simulink model "main_sim"  (R2025b)
settings: Solver=VariableStepAuto  StartTime=0.0  StopTime=6  RelTol=1e-3
model workspace (MAT data in the model file):
  Axy = [0  0  0  0; 0  0  0  0; 0  0  0  0; 0  0  0  0]
  Axz = [0  0  1  0; 0  0  0  1; 0  -11.8453251738  0  0; 0  6.95008459918  0  0]
  Ayz = [0  0  1  0; 0  0  0  1; 0  -11.8453251738  0  0; 0  6.95008459918  0  0]
  Bxy = [0  0  0  0; 0  0  0  0; 0  0  0  0; 0  0  0  0]
  Bxz = [0; 0; 9.84767991023; -1.08649077682]
  Byz = [0; 0; 9.84767991023; -1.08649077682]
  Cxy = [0  0  0  0; 0  0  0  0; 0  0  0  0; 0  0  0  0]
  Cxz = [1  0  0  0; 0  1  0  0; 0  0  1  0; 0  0  0  1]
  Cyz = [1  0  0  0; 0  1  0  0; 0  0  1  0; 0  0  0  1]
  Dxy = [0  0  0  0; 0  0  0  0; 0  0  0  0; 0  0  0  0]
  Dxz = [0; 0; 0; 0]
  Dyz = [0; 0; 0; 0]
  ICxy = [0; 0; 0; 0]
  ICxz = [0; 0.3; 0; -0.7]
  ICyz = [0; 0.3; 0; -0.7]
  ptorque = [0 0 0]
  vtorque = [0; 0; 0]
libraries: sim3dlib x7
settings Model: PacingRate=0.400000  Creator=rtsto  LastModifiedBy=rtsto

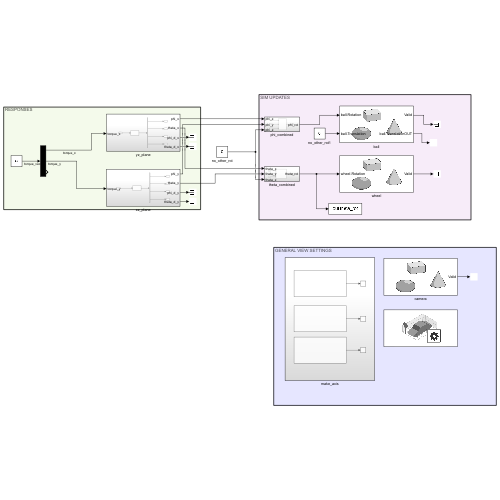
[thumbnail: Simulink's stored preview of the top-level diagram]
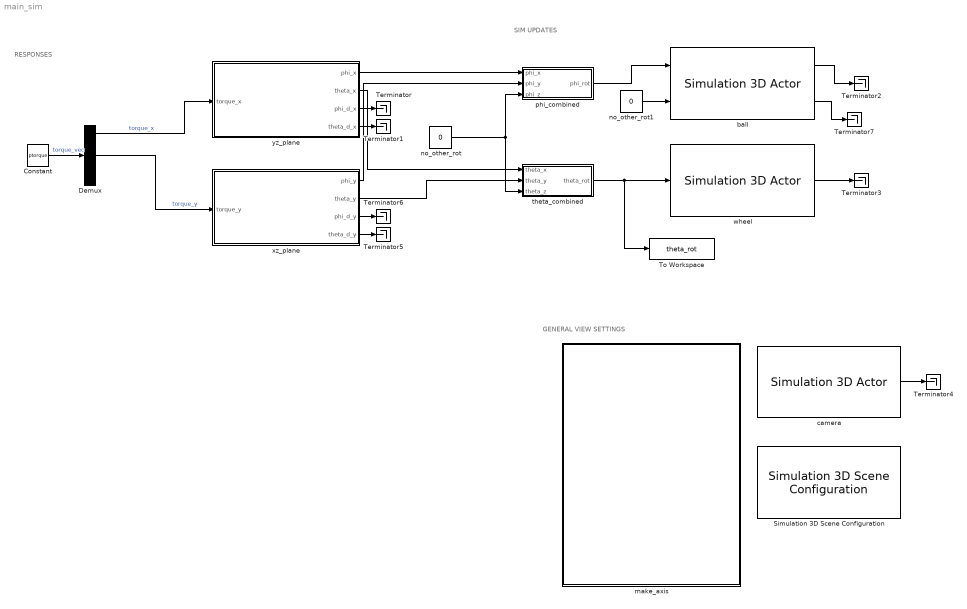
== system main_sim ==
  note: SIM UPDATES
  note: RESPONSES
  note: GENERAL VIEW SETTINGS
  Constant : Constant  Value=ptorque
  Demux : Demux  Outputs=3
  Simulation 3D Scene Configuration : sim3dlib/Simulation 3D Scene Configuration  Priority=0  ProjectFormat=Default Scenes  SceneDesc=Empty scene  ProjectName=C:\Program Files\MATLAB\R2025b\toolbox\shared\sim3d_projects\automotive_project_windows\UE\WindowsNoEditor\VehicleSimulation.exe  ScenePath=/Game/Maps/HwStrght  EnableOpenDRIVE=off  vehTagList={'Custom';'MainScene';'Scene Origin';'Viewpoint1';'World';'ball';'camera';'wheel';'x_axis';'y_axis';'z_axis'}  vehTag=MainScene  AttachedCameraRelativeTranslation=[0 0 0]  FreeCameraDefaultInitialTranslation=[-6, 0, 2]  AttachedCameraRelativeRotation=[0 0 0]  FreeCameraDefaultInitialRotation=[0, -15, 0]  ViewpointName=MainScene  FreeCameraInitialTranslation=[0 0 0]  ViewpointTranslation=[0 0 0]  FreeCameraInitialRotation=[0 0 0]  ViewpointRotation=[0 0 0]  OpVisEn=off  Ts=.02  EnableWindow=on  EnableRemoteAccess=off  EnableWeather=off  SunAzimuth=90  SunAltitude=40.0  EnableGeospatialSun=off  Latitude=0  Longitude=0  Date=2023-01-01  Time=10:30:00  GeoTimeZone=-5.0  SunDaylightSaving=off  wind=1  clouds=10  EnableVolumetricClouds=off  CloudCoverage=0  CloudAltitude=6  fog=0  rain=0  RaindropsEffect=off  SnowDensity=0  EnableGeospatial=off  TilesetSource=Earth terrain  UseTrueOrigin=off  OriginHeight=200  OriginLatitude=40.744652  OriginLongitude=-73.988864  MapStyle=Aerial  AdditionalAssetIDs=[]  UseAdvancedSunSky=off  SolarTime=11  TimeZone=-5  Day=21  Month=9  Year=2022  UseDaylightSavingTime=on  DSTStartDay=10  DSTStartMonth=3  DSTEndDay=3  DSTEndMonth=11  DSTSwitchHour=2  sensorTag=MainCamera1  sensorId=1  sensorName=MainCamera1  mountLoc=Origin  offsetFlag=off  tmountOffset=[0, 0, 0]  rmountOffset=[0, 0, 0]  HorizontalResolution=1280  VerticalResolution=720  HorizontalFOV=60  mountPoint=[0 0 0]  mountOrientation=[0 0 0]  aMode=5  ID=1  GeoTrigger=Inactive  ViewNameList={'Custom', 'World', 'MainScene', 'Viewpoint1'}  ViewTranslationList="{'[0 0 0]', '[0 0 0]', '[0 0 0]', '[-4  4  2]'}"  ViewRotationList="{'[0 0 0]', '[0 0 0]', '[0 0 0]', '[0        -22.5          -45]'}"
      settings: LibrarySourceBlock=sl3dlib/Simulation 3D/Environment/Simulation 3D Scene Configuration
  Terminator{,1..7} (8 alike) : Terminator
  To Workspace : ToWorkspace  VariableName=theta_rot  SampleTime=-1
  ball : sim3dlib/Simulation 3D Actor  Priority=1  ActorName=ball  ParentName=Scene Origin  Operation=Create at setup  InitScriptText=|  SampleTime=-1  Translation=single([0 0 0])  Rotation=single([0 0 0])  Scale=single([1 1 1])  InputsText=ball.Rotation ball.Translation  OutputsText=ball.Translation  aMode=5  ActorTag=ball  ActorType=Sim3dActor  ID=C
      | % BALL LOADING
      |     ball = sim3d.Actor(ActorName='ball', ...
      |         Mobility=sim3d.utils.MobilityTypes.Movable);
      |     load(ball, "ball.stl");
      |     diameter = 12.5; % raw
      |     scale = 0.1; % raw
      |     
      |     radius = scale*diameter/2; %scaled
      |     ball.Scale = scale*[1, 1, 1]; % NOTE: won't change in 'transform' tab
      |     ball.Translation = [0 -radius -radius];
      |     ball.Rotation = [0, pi/2, -pi/2]; % rad
      |     
      |     ball.Physics = false;
      |     ball.Collisions = true;
      |     
      |     ball.Color = [1 0 0];
      |     ball.Metallic = 0.1; % not at all
      |     ball.Shininess = 0; % not at all
      |     World.add(ball, Actor);
  camera : sim3dlib/Simulation 3D Actor  Priority=1  ActorName=camera  ParentName=Scene Origin  Operation=Create at setup  InitScriptText=|  SampleTime=-1  Translation=[0 0 0]  Rotation=[0 0 0]  Scale=[1 1 1]  aMode=5  ActorTag=camera  ActorType=Sim3dActor  ID=C
      | pos = [-4, 4, 2];
      | rot = [0, -22.5*pi/180, -45*pi/180];
      | camera = createViewport(World, ...
      |     Translation=pos, Rotation=rot);
  make_axis : Subsystem
  no_other_rot : Constant  Value=0  OutDataTypeStr=Inherit: Inherit via back propagation
  no_other_rot1 : Constant  Value=0  OutDataTypeStr=Inherit: Inherit via back propagation
  phi_combined : Subsystem
  theta_combined : Subsystem
  wheel : sim3dlib/Simulation 3D Actor  Priority=1  ActorName=wheel  ParentName=Scene Origin  Operation=Create at setup  InitScriptText=|  SampleTime=-1  Translation=single([0 0 0])  Rotation=single([0 0 0])  Scale=single([1 1 1])  InputsText=wheel.Rotation  aMode=5  ActorTag=wheel  ActorType=Sim3dActor  ID=C
      | % WHEEL LOADING
      | wheel = sim3d.Actor(ActorName='wheel', ...
      |     Mobility=sim3d.utils.MobilityTypes.Movable);
      | load(wheel, "ball.stl");
      | d = 12.5; % raw diameter, both
      | sw = 0.07; % raw scale, wheel
      | sb = 0.1; % raw scale, ball
      | 
      | rw = d*sw/2;
      | additional = (sb-sw)*(d/2);
      | wheel.Scale = sw*[1 1 1];
      | wheel.Translation = [additional, -rw, rw+additional];
      | wheel.Rotation = [0, pi/2, -pi/2]; %rad
      | 
      | wheel.Physics = false;
      | wheel.Collisions = false;
      | wheel.Gravity = false;
      | 
      | wheel.Color = [0 1 0];
      | wheel.Metallic = 0; % not at all
      | wheel.Shininess = 0; % not at all
      | 
      | World.add(wheel, Actor);
  xz_plane : Subsystem
  yz_plane : Subsystem
  wires:
  ball/1 -> Terminator2/1
  wheel/1 -> Terminator3/1
  phi_combined/1(phi_rot) -> ball/1
  yz_plane/3(phi_d_x) -> Terminator/1
  yz_plane/4(theta_d_x) -> Terminator1/1
  theta_combined/1(theta_rot) -> To Workspace/1, wheel/1
  yz_plane/1(phi_x) -> phi_combined/1(phi_x)
  yz_plane/2(theta_x) -> theta_combined/1(theta_x)
  no_other_rot/1 -> phi_combined/3(phi_z), theta_combined/3(theta_z)
  camera/1 -> Terminator4/1
  xz_plane/4(theta_d_y) -> Terminator5/1
  xz_plane/3(phi_d_y) -> Terminator6/1
  Constant/1 -> Demux/1  "torque_vec"
  Demux/1 -> yz_plane/1(torque_x)  "torque_x"
  Demux/2 -> xz_plane/1(torque_y)  "torque_y"
  xz_plane/1(phi_y) -> phi_combined/2(phi_y)
  xz_plane/2(theta_y) -> theta_combined/2(theta_y)
  ball/2 -> Terminator7/1
  no_other_rot1/1 -> ball/2

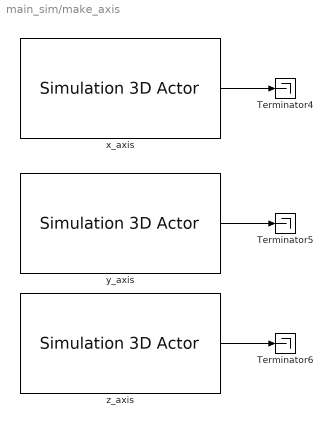
== system main_sim/make_axis ==
  Terminator4 : Terminator
  Terminator5 : Terminator
  Terminator6 : Terminator
  x_axis : sim3dlib/Simulation 3D Actor  Priority=1  ActorName=x_axis  ParentName=Scene Origin  Operation=Create at setup  InitScriptText=|  SampleTime=-1  Translation=[0 0 0]  Rotation=[0 0 0]  Scale=[1 1 1]  aMode=5  ActorTag=x_axis  ActorType=Sim3dActor  ID=C
      | xA = sim3d.Actor(ActorName='xA');
      | 
      | xA.createShape('box', [5 0.02 0.02]);
      | xA.Color = [1, 0, 0];
      | 
      | World.add(xA, Actor);
  y_axis : sim3dlib/Simulation 3D Actor  Priority=1  ActorName=y_axis  ParentName=Scene Origin  Operation=Create at setup  InitScriptText=|  SampleTime=-1  Translation=[0 0 0]  Rotation=[0 0 0]  Scale=[1 1 1]  aMode=5  ActorTag=y_axis  ActorType=Sim3dActor  ID=C
      | yA = sim3d.Actor(ActorName='yA');
      | 
      | yA.createShape('box', [0.02, 5, 0.02]);
      | yA.Color = [0, 1, 0];
      | 
      | World.add(yA, Actor);
  z_axis : sim3dlib/Simulation 3D Actor  Priority=1  ActorName=z_axis  ParentName=Scene Origin  Operation=Create at setup  InitScriptText=|  SampleTime=-1  Translation=[0 0 0]  Rotation=[0 0 0]  Scale=[1 1 1]  aMode=5  ActorTag=z_axis  ActorType=Sim3dActor  ID=C
      | zA = sim3d.Actor(ActorName='zA');
      | 
      | zA.createShape('box', [0.02, 0.02, 5]);
      | zA.Color = [0, 0, 1];
      | 
      | World.add(zA, Actor);
  wires:
  x_axis/1 -> Terminator4/1
  y_axis/1 -> Terminator5/1
  z_axis/1 -> Terminator6/1

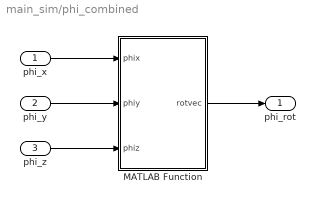
== system main_sim/phi_combined ==
  phi_x : Inport
  phi_y : Inport  Port=2
  phi_z : Inport  Port=3
  MATLAB Function : MATLAB Function  TreatAsAtomicUnit=on
  phi_rot : Outport
  wires:
  phi_x/1 -> MATLAB Function/1(phix)
  MATLAB Function/1(rotvec) -> phi_rot/1
  phi_y/1 -> MATLAB Function/2(phiy)
  phi_z/1 -> MATLAB Function/3(phiz)

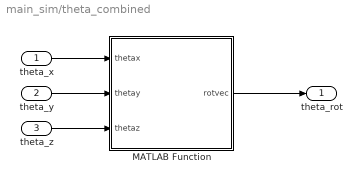
== system main_sim/theta_combined ==
  theta_x : Inport
  theta_y : Inport  Port=2
  theta_z : Inport  Port=3
  MATLAB Function : MATLAB Function  TreatAsAtomicUnit=on
  theta_rot : Outport
  wires:
  theta_x/1 -> MATLAB Function/1(thetax)
  theta_y/1 -> MATLAB Function/2(thetay)
  theta_z/1 -> MATLAB Function/3(thetaz)
  MATLAB Function/1(rotvec) -> theta_rot/1

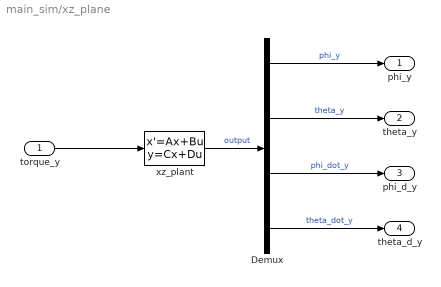
== system main_sim/xz_plane ==
  torque_y : Inport
  Demux : Demux
  xz_plant : StateSpace  A=Axz  B=Bxz  C=Cxz  D=Dxz  InitialCondition=ICxz
  phi_y : Outport
  theta_y : Outport  Port=2
  phi_d_y : Outport  Port=3
  theta_d_y : Outport  Port=4
  wires:
  xz_plant/1 -> Demux/1  "output"
  Demux/1 -> phi_y/1  "phi_y"
  Demux/2 -> theta_y/1  "theta_y"
  Demux/3 -> phi_d_y/1  "phi_dot_y"
  Demux/4 -> theta_d_y/1  "theta_dot_y"
  torque_y/1 -> xz_plant/1

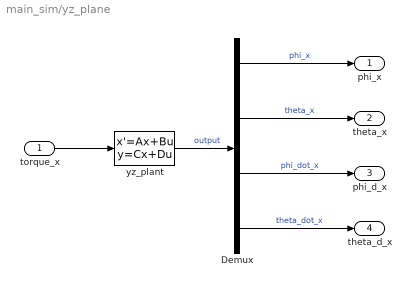
== system main_sim/yz_plane ==
  torque_x : Inport
  Demux : Demux
  yz_plant : StateSpace  A=Ayz  B=Byz  C=Cyz  D=Dyz  InitialCondition=ICyz
  phi_x : Outport
  theta_x : Outport  Port=2
  phi_d_x : Outport  Port=3
  theta_d_x : Outport  Port=4
  wires:
  torque_x/1 -> yz_plant/1
  yz_plant/1 -> Demux/1  "output"
  Demux/1 -> phi_x/1  "phi_x"
  Demux/2 -> theta_x/1  "theta_x"
  Demux/3 -> phi_d_x/1  "phi_dot_x"
  Demux/4 -> theta_d_x/1  "theta_dot_x"

== matlab function main_sim/phi_combined/MATLAB Function ==
  data: phix input; rotvec output; phiy input; phiz input
function rotvec = fcn(phix, phiy, phiz)


rotvec = reshape([phix; phiy; phiz], [1, 3]);

== matlab function main_sim/theta_combined/MATLAB Function ==
  data: thetax input; rotvec output; thetay input; thetaz input
function rotvec = fcn(thetax, thetay, thetaz)


rotvec = reshape([thetax; thetay; thetaz], [1, 3]);
